simulink model "MPPT_PSO"  (R2022a)
settings: Solver=FixedStepAuto  StartTime=0.0  StopTime=10  FixedStep=4e-6  RelTol=1e-3
libraries: spsSeriesRLCBranchLib x4, spsDiodeLib x2, spsCurrentMeasurementLib x1, spsMosfetLib x1, spsPVArrayLib x1, spsPWMGeneratorDCDCLib x1, spsVoltageMeasurementLib x1, spspowerguiLib x1
settings Model: Creator=ACER  LastModifiedBy=Thanh Quang
settings DataIOCC: ReturnWorkspaceOutputs=off
settings DebuggingCC: UnconnectedInputMsg=warning  UnconnectedOutputMsg=warning  UnconnectedLineMsg=warning  PregeneratedLibrarySubsystemCodeDiagnostic=none  SFMachineParentedDataDiag=warning  ArithmeticOperatorsInVariantConditions=warning
settings SFSimCC: SimUseLocalCustomCode=off  CustomCodeUndefinedFunction=UseInterfaceOnly
settings RTWCC: RTWUseLocalCustomCode=off

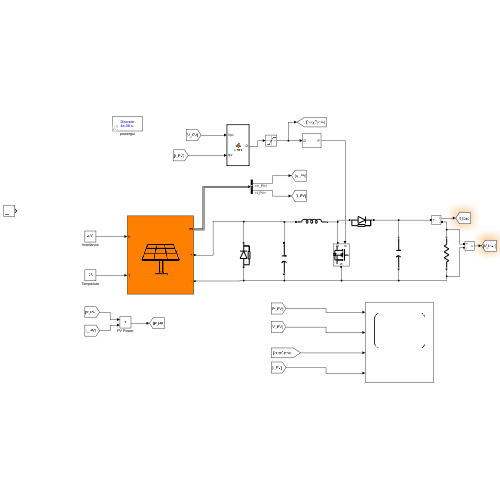
[thumbnail: Simulink's stored preview of the top-level diagram]
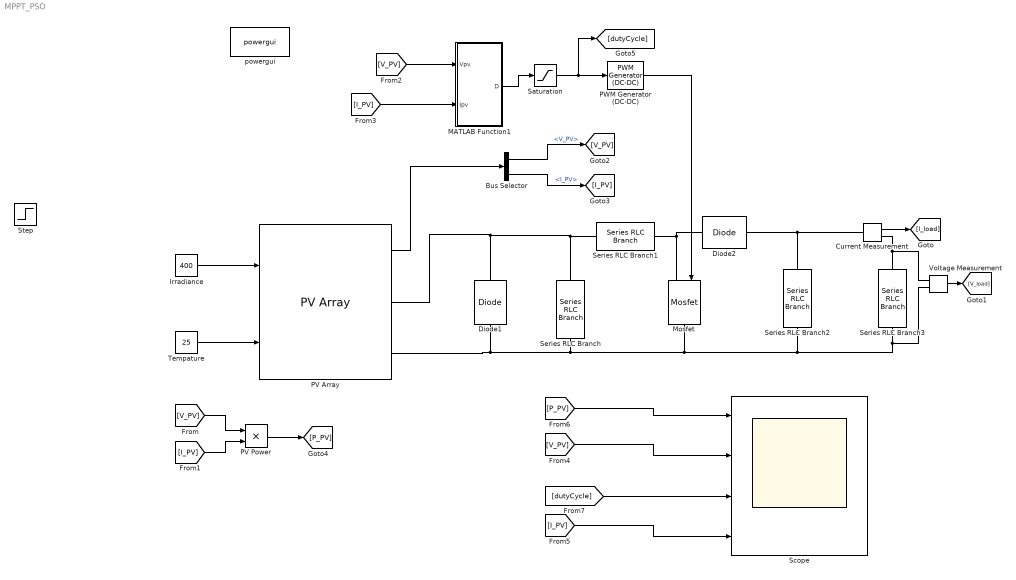
== system MPPT_PSO ==
  Bus Selector : BusSelector  OutputSignals=V_PV,I_PV
  Current Measurement : spsCurrentMeasurementLib/Current Measurement  PhasorSimulation=off  OutputType=Complex  PSBequivalent=0
  Diode1 : spsDiodeLib/Diode  Ron=0.001  Lon=0  Vf=0.8  IC=0  UseSnubber=0  Rs=500  Cs=250e-9  Measurements=off
  Diode2 : spsDiodeLib/Diode  Ron=0.001  Lon=0  Vf=0.8  IC=0  UseSnubber=0  Rs=500  Cs=250e-9  Measurements=off
  Irradiance : Constant  Value=400  SampleTime=4e-6
  MATLAB Function1 : MATLAB Function  TreatAsAtomicUnit=on
  Mosfet : spsMosfetLib/Mosfet  Ron=1e-3  Lon=0  Rd=1e-3  Vfd=0  IC=0  Rs=inf  Cs=inf  Measurements=off
  PV Array : spsPVArrayLib/PV Array  Npar=1  Nser=1  PlotType=array @ 25 deg.C & specified irradiances  S_vec="[ 1000  400 ]"  Temp_C_vec="[ 45 25  ]"  ModuleName=User-defined  PlotWhenSelected=off  Pm=248.977  Ncell=60  Voc=38.4  Isc=8.85  Vm=30.7  Im=8.11  beta_Voc_pc=-0.35599  alpha_Isc_pc=0.07  beta_Voc=-0.1367  alpha_Isc=0.006195  IL=8.8816  I0=2.622e-10  nI=1.0292  Rsh=104.8955  Rs=0.37421  RobustModel=off  RobustCellTemperature=313.3991  BAL=off  Tc=1e-6  Tfilter=4e-6
  PV Power : Product
  PWM Generator (DC-DC) : spsPWMGeneratorDCDCLib/PWM Generator (DC-DC)  Fsw=5000  Ts=4e-6
  Saturation : Saturate  UpperLimit=1  LowerLimit=0
  Scope : Scope  NumInputPorts=4
  Series RLC Branch : spsSeriesRLCBranchLib/Series RLC Branch  LConnTagsString=__new0  RConnTagsString=__new0  BranchType=C  Resistance=1  Inductance=1e-3  SetiL0=off  InitialCurrent=0  Capacitance=5e-3  Setx0=off  InitialVoltage=0  Measurements=None
  Series RLC Branch1 : spsSeriesRLCBranchLib/Series RLC Branch  LConnTagsString=__new0  RConnTagsString=__new0  BranchType=L  Resistance=1  Inductance=2.5e-3  SetiL0=off  InitialCurrent=0  Capacitance=1e-3  Setx0=off  InitialVoltage=0  Measurements=None
  Series RLC Branch2 : spsSeriesRLCBranchLib/Series RLC Branch  LConnTagsString=__new0  RConnTagsString=__new0  BranchType=C  Resistance=1  Inductance=1e-3  SetiL0=off  InitialCurrent=0  Capacitance=250e-6  Setx0=off  InitialVoltage=0  Measurements=None
  Series RLC Branch3 : spsSeriesRLCBranchLib/Series RLC Branch  LConnTagsString=__new0  RConnTagsString=__new0  BranchType=R  Resistance=30  Inductance=1e-3  SetiL0=off  InitialCurrent=0  Capacitance=1e-3  Setx0=off  InitialVoltage=0  Measurements=None
  Step : Step  Time=4  Before=400  After=1000  SampleTime=0
  Tempature : Constant  Value=25
  Voltage Measurement : spsVoltageMeasurementLib/Voltage Measurement  PhasorSimulation=off  OutputType=Complex  PSBequivalent=0
  powergui : spspowerguiLib/powergui  Priority=1  SimulationMode=Discrete  SampleTime=4e-6  frequency=60  Iterations=50  frequencyindice=0  Pbase=100e6  ErrMax=1e-4  UnitsV=kV  UnitsW=MW  buscounter=0  FunctionMessages=off  echomessages=off  EnableUseOfTLC=off  CurrentSourceSwitches=off  DisableSnubberDevices=off  DisableRonSwitches=off  DisableVfSwitches=off  DisplayEquations=off  AutomaticDiscreteSolvers=off  SolverType=Tustin/Backward Euler (TBE)  Interpol=off  ExternalGateDelay=off  methode=off  Ts=100  x0status=blocks  SPID=on  SwTol=0  HookPort=off  NonlinearTolerance=0  nMaxIteration=15  ContinueOnMaxIteration=off  RestoreLinks=warning  ResistiveCurrentMeasurement=off  Frange=[0:2:500]  Ylog=off  Xlog=on  ShowGrid=off  save=off  variable=ZData  structure=0  ZoomFFT=off  StartTime=0.0  cycles=1  DisplayStyle=1  fundamental=60  FreqAxis=off  MaxFrequency=1000  frequencyindicesteady=1  RmsSteady=1  display=off
  wires:
  Tempature/1 -> PV Array/2
  Current Measurement/1 -> [I_load]
  Voltage Measurement/1 -> [V_load]
  PV Array/1 -> Bus Selector/1
  Bus Selector/1 -> [V_PV]  "<V_PV>"
  Bus Selector/2 -> [I_PV]  "<I_PV>"
  [I_PV] -> PV Power/2
  [V_PV] -> PV Power/1
  PV Power/1 -> [P_PV]
  Saturation/1 -> [dutyCycle], PWM Generator (DC-DC)/1
  PWM Generator (DC-DC)/1 -> Mosfet/1
  [V_PV] -> Scope/2
  [P_PV] -> Scope/1
  [dutyCycle] -> Scope/3
  [I_PV] -> Scope/4
  MATLAB Function1/1(D) -> Saturation/1
  [V_PV] -> MATLAB Function1/1(Vpv)
  [I_PV] -> MATLAB Function1/2(Ipv)
  Irradiance/1 -> PV Array/1
  connections:
  PV Array/RConn1 -- Series RLC Branch/LConn1 -- Series RLC Branch1/LConn1 -- Diode1/RConn1
  PV Array/RConn2 -- Voltage Measurement/LConn2 -- Series RLC Branch3/RConn1 -- Series RLC Branch2/RConn1 -- Mosfet/RConn1 -- Series RLC Branch/RConn1 -- Diode1/LConn1
  Diode2/LConn1 -- Series RLC Branch1/RConn1 -- Mosfet/LConn1
  Diode2/RConn1 -- Current Measurement/LConn1 -- Series RLC Branch2/LConn1
  Current Measurement/RConn1 -- Voltage Measurement/LConn1 -- Series RLC Branch3/LConn1

== matlab function MPPT_PSO/MATLAB Function1 ==
  settings: updateMethod=DISCRETE
  data: Vpv input; D output; Ipv input
function D = PSO(Vpv,Ipv)
%%%CHECKEDDDDDD%%%%%%
persistent u;%u-th particle
persistent dcurrent;%store current duty cycle
persistent pbest;%store local best dc for power
persistent p;%  power for each particle
persistent dc;%store duty cycle ~ position 
persistent v;%velocity
persistent counter;%delay iteration
persistent gbest;%store global best dc for power
persistent convergence;%check dc convergence status
persistent P_prev;%store previous power
%initialization
num_agency = 3;
if(isempty(counter))
    counter = 0;
    dcurrent=0.5;
    gbest=0.9;
    p = zeros(num_agency,1);
    v=zeros(num_agency,1);
    pbest = zeros(num_agency,1);
    u=0;
    dc=zeros(num_agency,1);
    dc(1)=0.05;
    dc(2)=0.4;
    dc(3)=0.8;
    P_prev = Ipv*Vpv;
    convergence = 0;
end
if(convergence == 1)
        if(abs(Vpv*Ipv-P_prev)/(P_prev + 0.0001) >= 0.3)
            counter = 0;
            dcurrent=0.5;
            gbest=0.9;
            p = zeros(num_agency,1);
            v=zeros(num_agency,1);
            pbest = zeros(num_agency,1);
            u=0;
            dc=zeros(num_agency,1);
            convergence = 0;
            dc(1)=0.05;
            dc(2)=0.65;
            dc(3)=0.8;
        end
end
%%3800
if(counter >=1 && counter < 4000)
    D=dcurrent;
    counter= counter+1;
    return;
end

if(u>=1 && u<= num_agency)
    if((Vpv*Ipv)>p(u))
        p(u) = Vpv*Ipv;
        pbest(u)=dcurrent;
    end
end
u=u+1;
if(u==num_agency+2)
    u=1;
end
if(u>=1 && u<= num_agency)
    D=dc(u);    
    dcurrent=D;
    counter=1;
    return;
elseif(u==num_agency+1)
    [~,i]=max(p);
    gbest=pbest(i);
    D=gbest;
    dcurrent=D;
    counter=1;
    for i=1:num_agency
     v(i)=updatevelocity(v(i),pbest(i),dc(i),gbest);
      dc(i)=updateduty(dc(i),v(i));
    end 
     P_prev = Ipv*Vpv;
    convergence = checkconvergence(dc(1),dc(2),dc(3));
    return;
    
else
    D=0.5
end
end

function vfinal=updatevelocity(velocity,pobest,d,gwbest)

w=0.1;
c1=1.2;
c2=1.2;

vfinal = (w*velocity)+(c1*rand(1)*(pobest-d))+(c2*rand(1)*(gwbest-d));
end
function status = checkconvergence(d1,d2,d3)
    status = 0;
    rate = 0.05;
    if(abs(d1-d2) < rate)
        if(abs(d1-d3) < rate)
            if(abs(d2-d3) < rate)
                status = 1;
            end
        end
    end
end
function dfinal=updateduty(d,velocity)
dup=d+velocity;
if(dup>1)
    dfinal=1;
elseif(dup<0.1)
    dfinal=0,1;
else
    dfinal=dup;
end
end
